simulink library "gmt_Simulink"  (R2025a)
settings: Solver=VariableStepAuto  StartTime=0.0  StopTime=10.0  RelTol=1e-3
undefined symbols (not defined in the file or in its folder): Motor
settings Model: Creator=jmp8430  LastModifiedBy=jmp8430

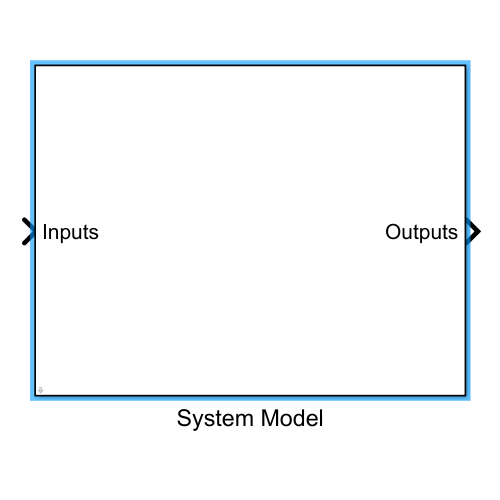
[thumbnail: Simulink's stored preview of the top-level diagram]
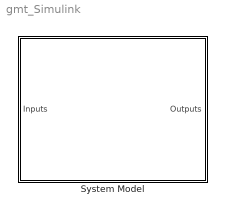
== system gmt_Simulink ==
  System Model : Subsystem  mask{GraphModelObj=Motor}
      mask prompts: GraphModelObj "Workspace Object"
      mask DialogControl DescGroupVar Prompt: Graph-Based Model Toolbox Simulink Block
      mask DialogControl DescTextVar Prompt: Mask automate the process to create a simulink block from a graph-based model toolbox function file output
      mask DialogControl ParameterGroupVar Prompt: Graph Model Input

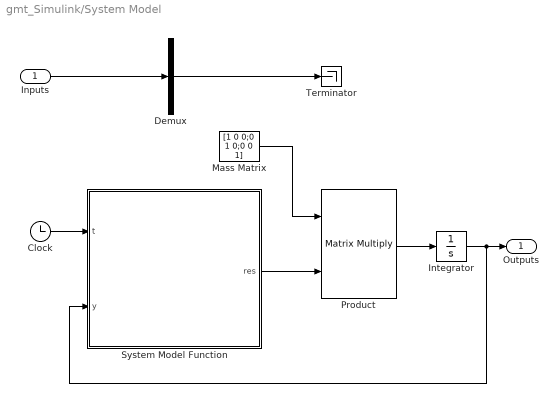
== system gmt_Simulink/System Model ==
  Inputs : Inport
  Clock : Clock
  Demux : Demux  Outputs=1
  Integrator : Integrator  InitialCondition=[1 1 1]'
  Mass Matrix : Constant  Value=[1 0 0;0 1 0;0 0 1]
  Product : Product  Multiplication=Matrix(*)
  System Model Function : MATLAB Function  TreatAsAtomicUnit=on
  Terminator : Terminator
  Outputs : Outport
  wires:
  Clock/1 -> System Model Function/1(t)
  Inputs/1 -> Demux/1
  Demux/1 -> Terminator/1
  Mass Matrix/1 -> Product/1
  System Model Function/1(res) -> Product/2
  Integrator/1 -> System Model Function/2(y), Outputs/1
  Product/1 -> Integrator/1

== matlab function gmt_Simulink/System Model/System Model Function ==
  data: t input; res output size=[3 1]; y input
% Code-Auto Generated By jmp8430 using gmt Toolbox on 14-Jan-2026 09:56:54
function res = sysFun_Motor(t,y)
J = 1;
Cp = 1;
L = 1;
b = 1;
c = 1;
R = 1;
Kt = 1;
x1 = y(1);
x2 = y(2);
x3 = y(3);
x1_dot = (1/(L*x1))*(-(Kt*x1*x2)-(R*x1^2));
x2_dot = (1/(J*x2))*(+(Kt*x1*x2)-(b*x2^2+c*x2));
x3_dot = (1/(Cp))*(+(b*x2^2+c*x2)+(R*x1^2));
res = [x1_dot;x2_dot;x3_dot];
end
